simulink model "predcstr"  (Simulink 7.1)
settings: Solver=ode45  SolverMode=SingleTasking  StartTime=0.0  StopTime=120  RelTol=1e-3  AbsTol=1e-6
undefined symbols (not defined in the file or in its folder): now, sfunxy2
settings Model: Creator=munlock -all d:\work\myr12\toolbox\fuzzy\fuzzy\mfedit.m  LastModifiedBy=Mark  ExtModeTrigMode=oneshot  ExtModeArmWhenConnect=off  TunableVars=prueba  TunableVarsStorageClass=Auto
settings DataIOCC: LimitDataPoints=off  SaveOutput=off  SignalLoggingName=sigsOut
settings OptimizationCC: BooleanDataType=off
settings DebuggingCC: SaveWithParameterizedLinksMsg=none  SignalResolutionControl=TryResolveAllWithWarning  SolverPrmCheckMsg=none  MultiTaskDSMMsg=warning  MultiTaskCondExecSysMsg=none  StrictBusMsg=None
settings HardwareCC: TargetUnknown=on
settings RTWCC: TemplateMakefile=grt_vc.tmf  IncludeERTFirstTime=on
settings GRTTargetCC: TargetFcnLib=ansi_tfl_tmw.mat

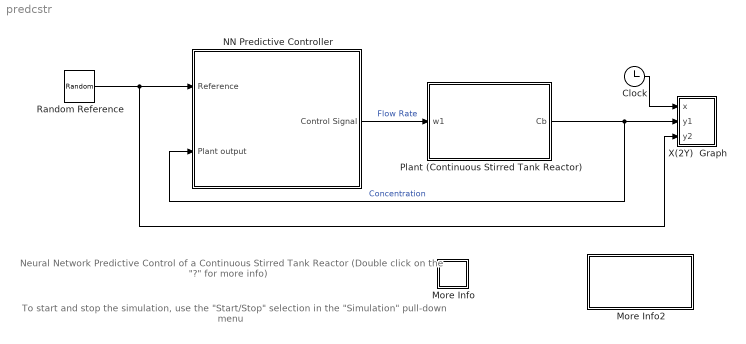
== system predcstr ==
  note: Neural Network Predictive Control of a Continuous Stirred Tank Reactor
      | (Double click on the "?" for more info)
  note: To start and stop the simulation, use the "Start/Stop"
      | selection in the "Simulation" pull-down menu
  Clock : Clock
      settings: Decimation=10
  More Info : Subsystem
      mask Display: disp('?')
  More Info2 : Subsystem
      settings: OpenFcn=simcad(bdroot)
      mask Display: disp('Double click\nhere for\nSimulink Help')
  NN Predictive Controller : Subsystem  mask(NN Predictive Controller){N2=7, Nu=2, Ts=0.2, rho=0.05, alpha=0.001, csrchfun=csrchbac, maxiter=2, S1=7, Ni=2, Nj=2, sim_file=cstr, trainfun=trainlm, Use_validation=1, Use_Testing=0, max_i=4, min_i=0, sam_training=8000, epochs=200, minp=0.02233575679015197, maxp=3.977181962055679, mint=19.990542740630676, maxt=23.003707300214998, Normalize=0, IW=[-20.531997924598212 18.706482494882994;0.0041681487931733516 -0.003898180117493663;0.0027271331329927679 -0.0026383962298670975;-4.2884263047654887 -2.5242458681173563;-7.5376751481296909 11.798966620249038;0.12631450792955951 0.63090781487873226;-9.0327138502332947 3.9557193990027328], LW1_2=[14.94314250694182 -17.959099344431603;-0.81834808440118445 0.41655850750692763;0.364433114947604 -0.17752308649608817;55.505918973874849 -51.271996485446365;-3.4857289415608221 2.5155674023943493;-1.0383681172774319 -0.1649807357299794;-1.7354318305331962 4.1593615744767991], LW2_1=[0.0026508898559841616 -1.0458797145936556 5.0292698388067745 0.00010141072535827776 0.0032962551987542432 0.58061299674354561 8.9082702971420182e-005], B1=[18.565258582766731;9.6542761594756836;-3.6577882481482806;-67.658021555936102;-2.7052627837062393;0.46399572090641622;-40.321245764315009], B2=21.149686119715415, max_i_int=20, min_i_int=5, limit_output=1, max_output=23, min_output=20, Use_Previous_Weights=1}
      mask prompts: Ts "Sample time"; rho "rho (typically = 0.03)"; alpha "alpha (typically = 0.001)"; csrchfun "Minimization rutine"; trainfun "Training function"
      mask help: NN Predictive Controller. You first train a neural network model of the plant to be controlled. The controller uses the plant model to predict plant performance over a specified time horizon. An optimization algorithm determines the control signal that optimizes plant performance over this horizon. Double click the NN Predictive Controller block to train the plant model and set the controller parameters.
      mask init:
      | xl = [0   .53   .53     .85   .85  .53  .53  NaN .85  .92 .92];
      | yl = [.95 .95 1.05  1.05   .82  .82  .95  NaN  .95 .95 .65];
      | x2 = [0 .53    NaN .92 1.2 NaN .53 .85 .85 .53 .53 ];
      | y2 = [.39 .39   NaN .65 .65 NaN .59 .59 .29 .29  .59];
      | x3 = [.67 .67 NaN .64 .67 .70 NaN .53 .4   .4   .53 NaN .46 .53 .46];
      | y3 = [.59 .82 NaN .66 .59 .66 NaN .55 .55 .86 .86 NaN  .89 .86 .83];
      | 
      | x1t=.03; y1t=.31;
      | x2t=.03; y2t=.8;
      | x8t=.03;y8t=.21;
      | x3t=.77; y3t=.53;
      | x4t=.77; y4t=.44;
      | x5t=.45; y5t=.76;
      | x6t=.45; y6t=.35;
      | x7t=.45; y7t=.25;
      settings: OpenFcn=nncontrolutil('nnpredict','',gcbh,gcb);
      mask StyleString: edit,edit,edit,edit,edit,popup(csrchgol|csrchbac|csrchhyb|csrchbre|csrchcha),edit,edit,edit,edit,edit,popup(trainbfg|trainbr |traincgb|traincgf|traincgp|traingd|traingdm|traingda|traingdx|trainlm |trainoss|trainrp |trainscg),edit,edit,edit,edit,edit,edit,edit,edit,edit,edit,edit,edit,edit,edit,edit,edit,edit,edit,edit,edit,edit,edit
      mask Display:
      | plot([[xl NaN x2]*.9-.075 ], [[yl  NaN y2]*.9-.1 ]);
      | plot([[x3]*.9-.075 ], [[y3]*.9-.1 ]);
      | text(x1t,y1t,'Plant');
      | text(x8t,y8t,'Output');
      | text(x2t,y2t,'Reference');
      | text(x3t,y3t,'Control');
      | text(x4t,y4t,'Signal');
      | text(x5t,y5t,'Optim.');
      | text(x6t,y6t,'NN');
      | text(x7t,y7t,'Model');
  Plant (Continuous Stirred Tank Reactor) : Subsystem  mask(Continuous Stirred Tank Reactor){}
      mask init:
      | xl = [0    .45  .45  NaN   .3   .3  1.   1.    NaN ];
      | yl = [1   1    .7    NaN   .8   .2    .2   .8  NaN  ]+.1;
      | x2 = [.85 .85   1.2   NaN .8 .85 .9 NaN .4 .45 .5 ];
      | y2 = [.7   1      1      NaN .8 .7   .8 NaN  .8 .7 .8]+.1;
      | x3 = [.3 1 NaN .8 .8 1.1 NaN 1 1.1 1];
      | y3 = [.6 .6 NaN .2 .1 .1 NaN .15 .1 .05]+.1;
      | t=(0:24)/24*2*pi;
      | xs = .07*cos(t)+.9;
      | ys = .07*sin(t)+.75;
      mask Display: plot([[xl NaN x2 NaN x3]*.9-.075 ], [[yl  NaN y2 NaN y3]*.9-.1 ]);
  Random Reference : UniformRandomNumber  Minimum=20  Maximum=23  Seed=round(now)  SampleTime=20
  X(2Y)  Graph : Subsystem  LoadFcn=sfunxy2([],[],[],'LoadBlock')  StartFcn=sfunxy2([],[],[],'Start')  StopFcn=sfunxy2([],[],[],'Stop')  mask(X(2Y) scope.){xmin=0, xmax=5, ymin=21, ymax=22, st=-1}
      mask prompts: xmin "x-min:"; xmax "x-max:"; ymin "y-min:"; ymax "y-max:"; st "Sample time:"
      mask help: X(2Y) scope using MATLAB graph window. First input is used as time base. Enter plotting ranges.
      settings: CopyFcn=sfunxy2([],[],[],'CopyBlock')  DeleteFcn=sfunxy2([],[],[],'DeleteBlock')  NameChangeFcn=sfunxy2([],[],[],'NameChange')
      mask Help: This block can be used to explore limit cycles. Look at the m-file sfunxy.m to see how it works.
      mask Display: plot([.05 .95 .95 .05 .05],[.45 .45 .95 .95 .45], 0.5+cos(0:0.1:2*pi)*0.3,0.7+sin(0:0.1:2*pi)*0.2)
  wires:
  Clock/1 -> X(2Y)  Graph/1(x)
  NN Predictive Controller/1(Control Signal) -> Plant (Continuous Stirred Tank Reactor)/1(w1)  "Flow Rate"
  Plant (Continuous Stirred Tank Reactor)/1(Cb) -> X(2Y)  Graph/2(y1), NN Predictive Controller/2(Plant output)  "Concentration"
  Random Reference/1 -> NN Predictive Controller/1(Reference), X(2Y)  Graph/3(y2)

== system predcstr/More Info ==
  note: This system simulates predictive control
      | of a continuous stirred tank reactor.
  note: Double-click on the NN Predictive Controller block
      | to set the controller parameters and train the plant model.
  note: For more information on what the controller
      | does, look under the mask of the NN Predictive
      | Controller block and look at the S-function p_opt2.m.

== system predcstr/More Info2 ==

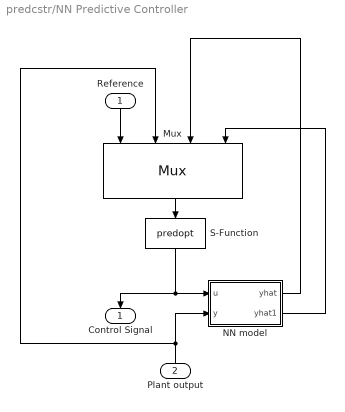
== system predcstr/NN Predictive Controller ==
  Reference : Inport  Orientation=down  OutDataType=sfix(16)  OutScaling=2^0
  Plant output : Inport  Orientation=up  Port=2  OutDataType=sfix(16)  OutScaling=2^0
  Mux : Mux  Orientation=down
      settings: DisplayOption=signals
  NN model : Subsystem
  S-Function : S-Function  Orientation=down  FunctionName=predopt  Parameters=N2,Ts,Nu,maxiter,csrchfun,rho,alpha,S1,IW,LW1_2,LW2_1,B1,B2,Ni,Nj,min_i,max_i,minp,maxp,mint,maxt,Normalize  EnableBusSupport=off
  Control Signal : Outport  Orientation=down  OutDataType=sfix(16)  OutScaling=2^0
  wires:
  Mux/1 -> S-Function/1
  S-Function/1 -> NN model/1(u), Control Signal/1
  NN model/2(yhat1) -> Mux/4
  NN model/1(yhat) -> Mux/3
  Reference/1 -> Mux/1
  Plant output/1 -> NN model/2(y), Mux/2

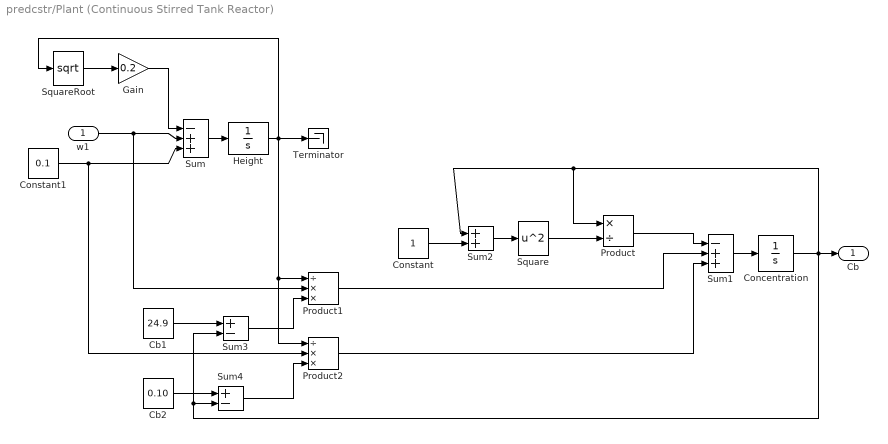
== system predcstr/Plant (Continuous Stirred Tank Reactor) ==
  w1 : Inport  OutDataType=sfix(16)  OutScaling=2^0
  Cb1 : Constant  Value=24.9  OutDataType=sfix(16)  OutScaling=2^0
  Cb2 : Constant  Value=0.10  OutDataType=sfix(16)  OutScaling=2^0
  Concentration : Integrator  InitialCondition=22  LowerSaturationLimit=0  ZeroCross=off
  Constant : Constant  OutDataType=sfix(16)  OutScaling=2^0
  Constant1 : Constant  Value=0.1  OutDataType=sfix(16)  OutScaling=2^0
  Gain : Gain  Gain=0.2  ParameterDataType=sfix(16)  ParameterScaling=2^0  OutDataType=sfix(16)  OutScaling=2^0  SaturateOnIntegerOverflow=on  OutDataTypeStr=Inherit: Same as input  ParamDataTypeStr=Inherit: Same as input
  Height : Integrator  InitialCondition=30  LimitOutput=on  LowerSaturationLimit=1  ZeroCross=off
  Product : Product  Inputs=*/  OutDataType=sfix(16)  OutScaling=2^0  SaturateOnIntegerOverflow=on  InputSameDT=on  OutDataTypeStr=Inherit: Same as first input
  Product1 : Product  Inputs=/**  OutDataType=sfix(16)  OutScaling=2^0  SaturateOnIntegerOverflow=on  InputSameDT=on  OutDataTypeStr=Inherit: Same as first input
  Product2 : Product  Inputs=/**  OutDataType=sfix(16)  OutScaling=2^0  SaturateOnIntegerOverflow=on  InputSameDT=on  OutDataTypeStr=Inherit: Same as first input
  Square : Math  Operator=square  OutDataType=sfix(16)  OutScaling=2^0  SaturateOnIntegerOverflow=on
  SquareRoot : Math  Operator=sqrt  OutDataType=sfix(16)  OutScaling=2^0  SaturateOnIntegerOverflow=on
  Sum : Sum  Inputs=-++  OutDataType=sfix(16)  OutScaling=2^0  SaturateOnIntegerOverflow=on  InputSameDT=on  OutDataTypeStr=Inherit: Same as first input
  Sum1 : Sum  Inputs=-++  OutDataType=sfix(16)  OutScaling=2^0  SaturateOnIntegerOverflow=on  InputSameDT=on  OutDataTypeStr=Inherit: Same as first input
  Sum2 : Sum  OutDataType=sfix(16)  OutScaling=2^0  SaturateOnIntegerOverflow=on  InputSameDT=on  OutDataTypeStr=Inherit: Same as first input
  Sum3 : Sum  Inputs=+-  OutDataType=sfix(16)  OutScaling=2^0  SaturateOnIntegerOverflow=on  InputSameDT=on  OutDataTypeStr=Inherit: Same as first input
  Sum4 : Sum  Inputs=+-  OutDataType=sfix(16)  OutScaling=2^0  SaturateOnIntegerOverflow=on  InputSameDT=on  OutDataTypeStr=Inherit: Same as first input
  Terminator : Terminator
  Cb : Outport  OutDataType=sfix(16)  OutScaling=2^0
  wires:
  Sum/1 -> Height/1
  Gain/1 -> Sum/1
  SquareRoot/1 -> Gain/1
  Height/1 -> SquareRoot/1, Product1/1, Product2/1, Terminator/1
  w1/1 -> Sum/2, Product1/2
  Constant1/1 -> Sum/3, Product2/2
  Cb1/1 -> Sum3/1
  Cb2/1 -> Sum4/1
  Sum3/1 -> Product1/3
  Sum4/1 -> Product2/3
  Concentration/1 -> Sum3/2, Sum4/2, Sum2/1, Product/1, Cb/1
  Constant/1 -> Sum2/2
  Sum2/1 -> Square/1
  Sum1/1 -> Concentration/1
  Square/1 -> Product/2
  Product/1 -> Sum1/1
  Product1/1 -> Sum1/2
  Product2/1 -> Sum1/3

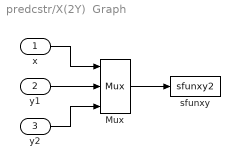
== system predcstr/X(2Y)  Graph ==
  x : Inport  OutDataType=sfix(16)  OutScaling=2^0
  y1 : Inport  Port=2  OutDataType=sfix(16)  OutScaling=2^0
  y2 : Inport  Port=3  OutDataType=sfix(16)  OutScaling=2^0
  Mux : Mux  Inputs=3
  sfunxy : S-Function  FunctionName=sfunxy2  Parameters=[xmin xmax ymin ymax], st  EnableBusSupport=off
  wires:
  y2/1 -> Mux/3
  y1/1 -> Mux/2
  x/1 -> Mux/1
  Mux/1 -> sfunxy/1

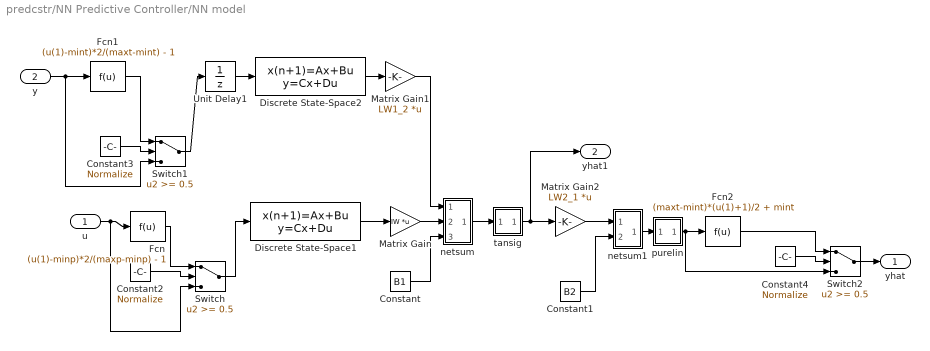
== system predcstr/NN Predictive Controller/NN model ==
  u : Inport  OutDataType=sfix(16)  OutScaling=2^0
  y : Inport  Port=2  OutDataType=sfix(16)  OutScaling=2^0
  Constant : Constant  Value=B1  OutDataType=sfix(16)  OutScaling=2^0
  Constant1 : Constant  Value=B2  OutDataType=sfix(16)  OutScaling=2^0
  Constant2 : Constant  Value=Normalize  OutDataType=sfix(16)  OutScaling=2^0
  Constant3 : Constant  Value=Normalize  OutDataType=sfix(16)  OutScaling=2^0
  Constant4 : Constant  Value=Normalize  OutDataType=sfix(16)  OutScaling=2^0
  Discrete State-Space1 : DiscreteStateSpace  A=[0 zeros(1,Ni-2);eye(Ni-2,Ni-1)]  B=[zeros(double(Ni==1));eye(Ni-1,1)]  C=[0 zeros(1,Ni-2);eye(Ni-1,Ni-1)]  D=eye(Ni,1)  SampleTime=Ts
  Discrete State-Space2 : DiscreteStateSpace  A=[0 zeros(1,Nj-2);eye(Nj-2,Nj-1)]  B=[zeros(double(Nj==1));eye(Nj-1,1)]  C=[0 zeros(1,Nj-2);eye(Nj-1,Nj-1)]  D=eye(Nj,1)  SampleTime=Ts
  Fcn : Fcn  Expr=(u(1)-minp)*2/(maxp-minp) - 1
  Fcn1 : Fcn  Expr=(u(1)-mint)*2/(maxt-mint) - 1
  Fcn2 : Fcn  Expr=(maxt-mint)*(u(1)+1)/2 + mint
  Matrix Gain : Gain  Gain=IW  Multiplication=Matrix(K*u)  ParameterDataType=sfix(16)  ParameterScaling=2^0  OutDataType=sfix(16)  OutScaling=2^0  SaturateOnIntegerOverflow=on  OutDataTypeStr=Inherit: Same as input  ParamDataTypeStr=Inherit: Same as input
  Matrix Gain1 : Gain  Gain=LW1_2  Multiplication=Matrix(K*u)  ParameterDataType=sfix(16)  ParameterScaling=2^0  OutDataType=sfix(16)  OutScaling=2^0  SaturateOnIntegerOverflow=on  OutDataTypeStr=Inherit: Same as input  ParamDataTypeStr=Inherit: Same as input
  Matrix Gain2 : Gain  Gain=LW2_1  Multiplication=Matrix(K*u)  ParameterDataType=sfix(16)  ParameterScaling=2^0  OutDataType=sfix(16)  OutScaling=2^0  SaturateOnIntegerOverflow=on  OutDataTypeStr=Inherit: Same as input  ParamDataTypeStr=Inherit: Same as input
  Switch : Switch  Threshold=0.5  ZeroCross=off  SaturateOnIntegerOverflow=on  InputSameDT=on
  Switch1 : Switch  Threshold=0.5  ZeroCross=off  SaturateOnIntegerOverflow=on  InputSameDT=on
  Switch2 : Switch  Threshold=0.5  ZeroCross=off  SaturateOnIntegerOverflow=on  InputSameDT=on
  Unit Delay1 : UnitDelay  SampleTime=Ts
  netsum : Subsystem
      mask Display: disp('+')
  netsum1 : Subsystem
      mask Display: disp('+')
  purelin : Subsystem
      mask Display: plot([-1 1],[0 0],[-1 1],[-1 1])
  tansig : Subsystem
      mask Display: plot([-1 1],[0 0],[-1 -.9 -.8 -.7 -.6 -.5 -.4 -.3 -.2 -.1 0 .1 .2 .3 .4 .5 .6 .7 .8 .9 1],2./(1+exp(-8*[-1 -.9 -.8 -.7 -.6 -.5 -.4 -.3 -.2 -.1 0 .1 .2 .3 .4 .5 .6 .7 .8 .9 1]))-1)
  yhat : Outport  OutDataType=sfix(16)  OutScaling=2^0
  yhat1 : Outport  Port=2  OutDataType=sfix(16)  OutScaling=2^0
  wires:
  netsum1/1(Out1) -> purelin/1(n)
  Constant1/1 -> netsum1/2(In2)
  Matrix Gain2/1 -> netsum1/1(In1)
  netsum/1(Out1) -> tansig/1(n)
  Constant/1 -> netsum/3(In3)
  Matrix Gain1/1 -> netsum/1(In1)
  Matrix Gain/1 -> netsum/2(In2)
  tansig/1(a) -> Matrix Gain2/1, yhat1/1
  Discrete State-Space1/1 -> Matrix Gain/1
  Fcn/1 -> Switch/1
  Switch/1 -> Discrete State-Space1/1
  u/1 -> Fcn/1, Switch/3
  Constant2/1 -> Switch/2
  Discrete State-Space2/1 -> Matrix Gain1/1
  Unit Delay1/1 -> Discrete State-Space2/1
  Constant3/1 -> Switch1/2
  Switch1/1 -> Unit Delay1/1
  Fcn1/1 -> Switch1/1
  y/1 -> Fcn1/1, Switch1/3
  Constant4/1 -> Switch2/2
  Switch2/1 -> yhat/1
  Fcn2/1 -> Switch2/1
  purelin/1(a) -> Fcn2/1, Switch2/3

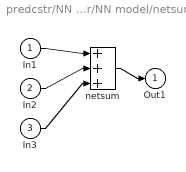
== system predcstr/NN Predictive Controller/NN model/netsum ==
  In1 : Inport  OutDataType=sfix(16)  OutScaling=2^0
  In2 : Inport  Port=2  OutDataType=sfix(16)  OutScaling=2^0
  In3 : Inport  Port=3  OutDataType=sfix(16)  OutScaling=2^0
  netsum : Sum  Inputs=3  OutDataType=sfix(16)  OutScaling=2^0  SaturateOnIntegerOverflow=on  InputSameDT=on  OutDataTypeStr=Inherit: Same as first input
  Out1 : Outport  OutDataType=sfix(16)  OutScaling=2^0
  wires:
  In1/1 -> netsum/1
  In2/1 -> netsum/2
  In3/1 -> netsum/3
  netsum/1 -> Out1/1

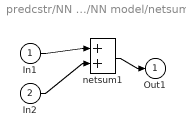
== system predcstr/NN Predictive Controller/NN model/netsum1 ==
  In1 : Inport  OutDataType=sfix(16)  OutScaling=2^0
  In2 : Inport  Port=2  OutDataType=sfix(16)  OutScaling=2^0
  netsum1 : Sum  Inputs=2  OutDataType=sfix(16)  OutScaling=2^0  SaturateOnIntegerOverflow=on  InputSameDT=on  OutDataTypeStr=Inherit: Same as first input
  Out1 : Outport  OutDataType=sfix(16)  OutScaling=2^0
  wires:
  In1/1 -> netsum1/1
  In2/1 -> netsum1/2
  netsum1/1 -> Out1/1

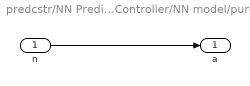
== system predcstr/NN Predictive Controller/NN model/purelin ==
  n : Inport  OutDataType=sfix(16)  OutScaling=2^0
  a : Outport  OutDataType=sfix(16)  OutScaling=2^0
  wires:
  n/1 -> a/1

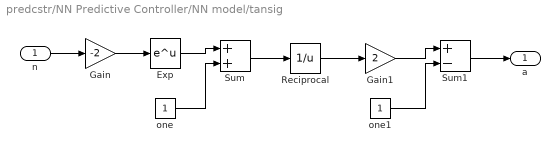
== system predcstr/NN Predictive Controller/NN model/tansig ==
  n : Inport  OutDataType=sfix(16)  OutScaling=2^0
  Exp : Math  OutDataType=sfix(16)  OutScaling=2^0  SaturateOnIntegerOverflow=on
  Gain : Gain  Gain=-2  ParameterDataType=sfix(16)  ParameterScaling=2^0  OutDataType=sfix(16)  OutScaling=2^0  SaturateOnIntegerOverflow=on  OutDataTypeStr=Inherit: Same as input  ParamDataTypeStr=Inherit: Same as input
  Gain1 : Gain  Gain=2  ParameterDataType=sfix(16)  ParameterScaling=2^0  OutDataType=sfix(16)  OutScaling=2^0  SaturateOnIntegerOverflow=on  OutDataTypeStr=Inherit: Same as input  ParamDataTypeStr=Inherit: Same as input
  Reciprocal : Math  Operator=reciprocal  OutDataType=sfix(16)  OutScaling=2^0  SaturateOnIntegerOverflow=on
  Sum : Sum  OutDataType=sfix(16)  OutScaling=2^0  SaturateOnIntegerOverflow=on  InputSameDT=on  OutDataTypeStr=Inherit: Same as first input
  Sum1 : Sum  Inputs=+-  OutDataType=sfix(16)  OutScaling=2^0  SaturateOnIntegerOverflow=on  InputSameDT=on  OutDataTypeStr=Inherit: Same as first input
  one : Constant  OutDataType=sfix(16)  OutScaling=2^0
  one1 : Constant  OutDataType=sfix(16)  OutScaling=2^0
  a : Outport  OutDataType=sfix(16)  OutScaling=2^0
  wires:
  n/1 -> Gain/1
  Gain/1 -> Exp/1
  Exp/1 -> Sum/1
  one/1 -> Sum/2
  Sum/1 -> Reciprocal/1
  Reciprocal/1 -> Gain1/1
  Gain1/1 -> Sum1/1
  one1/1 -> Sum1/2
  Sum1/1 -> a/1
